simulink model "ADAC_AEBS_FailOperationTest_A3_cs"  (R2014b)
settings: Solver=ode5  SolverMode=SingleTasking  StartTime=0.0  StopTime=inf  FixedStep=1/100  RelTol=1e-3
PreLoadFcn:
  | mbxruntime.callbacks.PreLoadFcn(bdroot);
  | check_NUTS_defined;
  | 
  | assignin('base',['model_closed_' bdroot],false);addpath('../includes_AEBS');
PostLoadFcn:
  | mbxruntime.callbacks.PostLoadFcn(bdroot);
InitFcn:
  | mbxruntime.callbacks.InitFcn(bdroot);
StartFcn:
  | mbxruntime.callbacks.StartFcn(bdroot);
StopFcn:
  | mbxruntime.callbacks.StopFcn(bdroot);
model workspace: external: MAT-File .\ADAC_AEBS_FailOperationTest_A3_cs_hws.mat (data not in the file)
undefined symbols (not defined in the file or in its folder): OrientationPitch, OrientationRoll, PositionX, PositionY, PositionZ, warningInitialVelocity, x0
undefined symbols (not defined in the file): ADAC_AEBS_FailOperationTest_A3_cs_022733f5fb7b020c, ADAC_AEBS_FailOperationTest_A3_cs_0e96c704d6d8ad21, ADAC_AEBS_FailOperationTest_A3_cs_160591024d30e51e, ADAC_AEBS_FailOperationTest_A3_cs_1af48b7bc7debef8, ADAC_AEBS_FailOperationTest_A3_cs_1c8862e820c7afdc, ADAC_AEBS_FailOperationTest_A3_cs_27e9254a11318684, ADAC_AEBS_FailOperationTest_A3_cs_34a9a7fc03d9473b, ADAC_AEBS_FailOperationTest_A3_cs_530c6f2a943bd468, ADAC_AEBS_FailOperationTest_A3_cs_591c8395df5aa215, ADAC_AEBS_FailOperationTest_A3_cs_7b366378d0e5b506, ADAC_AEBS_FailOperationTest_A3_cs_7d53398e9c5959a5, ADAC_AEBS_FailOperationTest_A3_cs_943491cbf915f302, ADAC_AEBS_FailOperationTest_A3_cs_9d3d862437c23341, ADAC_AEBS_FailOperationTest_A3_cs_b6ec93f5a18de3a7, ADAC_AEBS_FailOperationTest_A3_cs_e449793b2137b4b8, SteeringColumn, SteeringWheel, WheelL0, WheelL1, WheelR0, WheelR1
libraries: simulink_extras x33, simulink x21, PreScanSimulinkLibrary x5, PreScanUsefulBlocks x2
(part 1 of 10)
CloseFcn:
  | mbxruntime.callbacks.CloseFcn(bdroot);
  | evalin('base',['clear model_closed_' bdroot]);
settings Model: Creator=PRESCAN  LastModifiedBy=jenkins
settings DataIOCC: SignalLoggingSaveFormat=ModelDataLogs
settings OptimizationCC: InlineParams=on  ExpressionDepthLimit=2147483647  InitFltsAndDblsToZero=on
settings DebuggingCC: SaveWithParameterizedLinksMsg=none  UnderspecifiedInitializationDetection=Classic  MergeDetectMultiDrivingBlocksExec=none  SignalResolutionControl=TryResolveAllWithWarning  SolverPrmCheckMsg=none  MultiTaskDSMMsg=warning  MultiTaskCondExecSysMsg=none  FcnCallInpInsideContextMsg=UseLocalSettings  StateNameClashWarn=warning
settings ModelReferenceCC: UpdateModelReferenceTargets=IfOutOfDate
settings SFSimCC: SimParseCustomCode=off
settings SFSimCC: SimCustomHeaderCode=|
  | #include "prescan.h"
  | #include "prescan_platform.h"
settings RTWCC: IncludeERTFirstTime=on
settings GRTTargetCC: TargetFcnLib=ansi_tfl_tmw.mat  CombineOutputUpdateFcns=off  GRTInterface=on

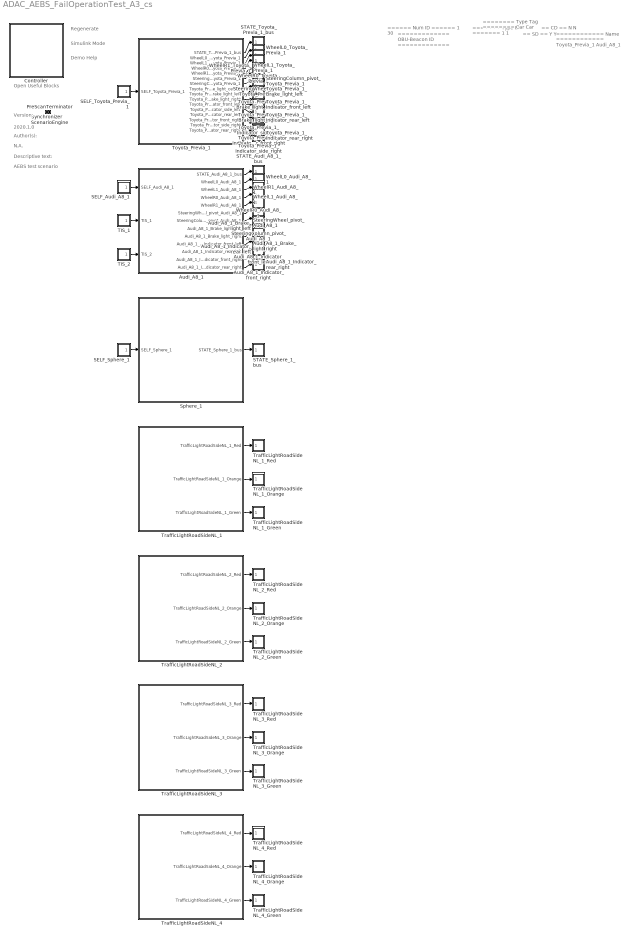
== system ADAC_AEBS_FailOperationTest_A3_cs ==
  note: Regenerate
  note: Simulink Mode
  note: Open Useful Blocks
  note: 2020.1.0
  note: Version:
  note: Author(s):
  note: N.A.
  note: Descriptive text:
  note: AEBS test scenario
  note: Demo Help
  note: ======
      | Num ID
      | ======
      | 1
      | 30
  note: =============
      | OBU-Beacon ID
      | =============
  note: =======
      | Type ID
      | =======
      | 1
      | 1
  note: ========
      | Type Tag
      | ========
      | Car
      | Car
  note: ==
      | SD
      | ==
      | Y
      | Y
  note: ==
      | CD
      | ==
      | N
      | N
  note: ============
      | Name
      | ============
      | Toyota_Previa_1
      | Audi_A8_1
  Audi_A8_1 : Subsystem  Tag=WorldObjectSubSystem  InitFcn=UniqueId = '69';
      mask init:
      | modelPath = GenericModelHelper.getGenericModelFilePath('ModelDepo','Vehicles\Audi_A8\Audi_A8.pgmb','e33fe1ddcf3e8ae97caccbc8f2fa74ac');imagePath = GenericModelHelper.getCompilationPicture(modelPath, 'Audi_A8_HighPoly.png');
      mask Display: image(imread(imagePath));color('white');text(0, 0, ' ID=30\n')
  Audi_A8_1_Brake_light_left : Subsystem  Tag=actuator/BrakeLightL  Priority=0  LoadFcn=load('PreScanVisuLightActuatorData');load('PrescanRPYData');load('PrescanXYZData');load('PreScanRGBData')  mask(PreScan Sink Block: VisuActiveLight){}
      mask help:
      | The VisuActiveLight block provides a way for detailed animation of Light Sources, such as the indicator, brake, fog and main lights of a vehicle, or a light post.
      |
      | For more information, please click Help.
      settings: OpenFcn=open_system([gcb '/Actuator'],'mask')
      mask Help: eval('openHelp(209)')
      mask Display: image(imread('HeadLight.png'))
  Audi_A8_1_Brake_light_right : Subsystem  Tag=actuator/BrakeLightR  Priority=0  LoadFcn=load('PreScanVisuLightActuatorData');load('PrescanRPYData');load('PrescanXYZData');load('PreScanRGBData')  mask(PreScan Sink Block: VisuActiveLight){}
      mask help:
      | The VisuActiveLight block provides a way for detailed animation of Light Sources, such as the indicator, brake, fog and main lights of a vehicle, or a light post.
      |
      | For more information, please click Help.
      settings: OpenFcn=open_system([gcb '/Actuator'],'mask')
      mask Help: eval('openHelp(209)')
      mask Display: image(imread('HeadLight.png'))
  Audi_A8_1_Indicator_front_left : Subsystem  Tag=actuator/IndicatorFL  Priority=0  LoadFcn=load('PreScanVisuLightActuatorData');load('PrescanRPYData');load('PrescanXYZData');load('PreScanRGBData')  mask(PreScan Sink Block: VisuActiveLight){}
      mask help:
      | The VisuActiveLight block provides a way for detailed animation of Light Sources, such as the indicator, brake, fog and main lights of a vehicle, or a light post.
      |
      | For more information, please click Help.
      settings: OpenFcn=open_system([gcb '/Actuator'],'mask')
      mask Help: eval('openHelp(209)')
      mask Display: image(imread('HeadLight.png'))
  Audi_A8_1_Indicator_front_right : Subsystem  Tag=actuator/IndicatorFR  Priority=0  LoadFcn=load('PreScanVisuLightActuatorData');load('PrescanRPYData');load('PrescanXYZData');load('PreScanRGBData')  mask(PreScan Sink Block: VisuActiveLight){}
      mask help:
      | The VisuActiveLight block provides a way for detailed animation of Light Sources, such as the indicator, brake, fog and main lights of a vehicle, or a light post.
      |
      | For more information, please click Help.
      settings: OpenFcn=open_system([gcb '/Actuator'],'mask')
      mask Help: eval('openHelp(209)')
      mask Display: image(imread('HeadLight.png'))
  Audi_A8_1_Indicator_rear_left : Subsystem  Tag=actuator/IndicatorRL  Priority=0  LoadFcn=load('PreScanVisuLightActuatorData');load('PrescanRPYData');load('PrescanXYZData');load('PreScanRGBData')  mask(PreScan Sink Block: VisuActiveLight){}
      mask help:
      | The VisuActiveLight block provides a way for detailed animation of Light Sources, such as the indicator, brake, fog and main lights of a vehicle, or a light post.
      |
      | For more information, please click Help.
      settings: OpenFcn=open_system([gcb '/Actuator'],'mask')
      mask Help: eval('openHelp(209)')
      mask Display: image(imread('HeadLight.png'))
  Audi_A8_1_Indicator_rear_right : Subsystem  Tag=actuator/IndicatorRR  Priority=0  LoadFcn=load('PreScanVisuLightActuatorData');load('PrescanRPYData');load('PrescanXYZData');load('PreScanRGBData')  mask(PreScan Sink Block: VisuActiveLight){}
      mask help:
      | The VisuActiveLight block provides a way for detailed animation of Light Sources, such as the indicator, brake, fog and main lights of a vehicle, or a light post.
      |
      | For more information, please click Help.
      settings: OpenFcn=open_system([gcb '/Actuator'],'mask')
      mask Help: eval('openHelp(209)')
      mask Display: image(imread('HeadLight.png'))
  Controller : Subsystem  Description=8A3CD2955739A82C886C20AE3E253D78460D53180EE2C1B14CC08DF75A70BE77  Priority=-1  LoadFcn=load PreScanControllerData  mask(PreScan Simulation Controller){prescanversion='2020.1.0', ModelReferencing=off, TimeStep=1/100, ControlMode=0, PreScanExecutionMode=on, ControllerCount=0, ControllerIndex=0, ControllerOptions=''}
      mask prompts: prescanversion "PreScan Version"; ModelReferencing "Use Model Referencing"; TimeStep "Upload Period [s]"; ControlMode "Control Mode"; PreScanExecutionMode "Execution Mode"; ControllerCount "Controller Count"; ControllerIndex "Controller Index"; ControllerOptions "Controller Options"
      mask help:
      | Please do not remove this block from the compilation sheet,
      | as it connects the model to the PreScan environment.
      mask init:
      | model = bdroot(gcb);
      | ExperimentFile = mbxruntime.findExperimentFile(model,true); %relative path
      | 
      | [d1, d2, d3, prescandata] = prescan_Settings();
      | ModelDepo = fullfile(prescandata,'ModelDepo'); 
      | 
      | RTmode = mbxruntime.getRTMode(model);
      | 
      | SimulationMode = get_param(bdroot,'SimulationMode');
      | if strcmp(SimulationMode, 'rapid-accelerator')
      |     SimulationMode = 'external';
      | end
      | TargetName = get_param(bdroot,'SystemTargetFile');
      settings: ModelCloseFcn=assignin('base',['model_closed_' bdroot],true);
      mask Help: eval('openHelp(812)')
      mask Display: image(imread('prescanlogo.ico'))
  PreScanTerminator : Subsystem  Tag=PreScanTerminator  Priority=999  LoadFcn=load PrescanTerminatorData  mask(PreScan Simulation Terminator){TimeStep=1/100}
      mask prompts: TimeStep "Upload Period [s]"
      mask help:
      | Please do not remove this block from the compilation sheet as it
      | connects the model to the PreScan environment.
      mask Help: eval('openHelp(812)')
      mask Display: image(imread('prescanlogo.ico'))
  SELF_Audi_A8_1 : Subsystem  Tag=sensor/SelfPort  Priority=30  LoadFcn=load('PreScanSelfSensorData.mat')  mask(PreScan Source Block: SELF){}
      mask help:
      | The SELF port shows (state) information of the actor itself. The outputs are position in the experiment's axis system and the GPS coordinates, and the object's absolute velocity and compass heading.
      |
      | For more information, please click Help.
      settings: OpenFcn=open_system([gcb '/Sensor'],'mask')
      mask Help: eval('openHelp(462)')
      mask Display: image(imread('GPS.png'))
  SELF_Sphere_1 : Subsystem  Tag=sensor/SelfPort  Priority=30  LoadFcn=load('PreScanSelfSensorData.mat')  mask(PreScan Source Block: SELF){}
      mask help:
      | The SELF port shows (state) information of the actor itself. The outputs are position in the experiment's axis system and the GPS coordinates, and the object's absolute velocity and compass heading.
      |
      | For more information, please click Help.
      settings: OpenFcn=open_system([gcb '/Sensor'],'mask')
      mask Help: eval('openHelp(462)')
      mask Display: image(imread('GPS.png'))
  SELF_Toyota_Previa_1 : Subsystem  Tag=sensor/SelfPort  Priority=30  LoadFcn=load('PreScanSelfSensorData.mat')  mask(PreScan Source Block: SELF){}
      mask help:
      | The SELF port shows (state) information of the actor itself. The outputs are position in the experiment's axis system and the GPS coordinates, and the object's absolute velocity and compass heading.
      |
      | For more information, please click Help.
      settings: OpenFcn=open_system([gcb '/Sensor'],'mask')
      mask Help: eval('openHelp(462)')
      mask Display: image(imread('GPS.png'))
  STATE_Audi_A8_1_bus : Subsystem  Tag=actuator/StatePort  Priority=0  LoadFcn=load('PreScanStateActuatorData.mat')  mask(PreScan Sink Block: State){}
      mask help:
      | The Actor State contains a vector signal of size (9x1), containing the following signals:
      |
      | -  Position    	(x,y,z)             	[m]
      | -  Velocity    	(vx,vy,vz)         	[m/s]
      | -  Angles       	(Roll, Pitch, Yaw)	[rad]
      |
      | The Actor state is defined in the global axis system.
      | The state is superponed on the Initial position defined in the GUI.
      |
      | For more information, please click Help.
      settings: OpenFcn=open_system([gcb '/Actuator'],'mask')
      mask Help: eval('openHelp(222)')
      mask Display: image(imread('State.png'))
  STATE_Sphere_1_bus : Subsystem  Tag=actuator/StatePort  Priority=0  LoadFcn=load('PreScanStateActuatorData.mat')  mask(PreScan Sink Block: State){}
      mask help:
      | The Actor State contains a vector signal of size (9x1), containing the following signals:
      |
      | -  Position    	(x,y,z)             	[m]
      | -  Velocity    	(vx,vy,vz)         	[m/s]
      | -  Angles       	(Roll, Pitch, Yaw)	[rad]
      |
      | The Actor state is defined in the global axis system.
      | The state is superponed on the Initial position defined in the GUI.
      |
      | For more information, please click Help.
      settings: OpenFcn=open_system([gcb '/Actuator'],'mask')
      mask Help: eval('openHelp(222)')
      mask Display: image(imread('State.png'))
  STATE_Toyota_Previa_1_bus : Subsystem  Tag=actuator/StatePort  Priority=0  LoadFcn=load('PreScanStateActuatorData.mat')  mask(PreScan Sink Block: State){}
      mask help:
      | The Actor State contains a vector signal of size (9x1), containing the following signals:
      |
      | -  Position    	(x,y,z)             	[m]
      | -  Velocity    	(vx,vy,vz)         	[m/s]
      | -  Angles       	(Roll, Pitch, Yaw)	[rad]
      |
      | The Actor state is defined in the global axis system.
      | The state is superponed on the Initial position defined in the GUI.
      |
      | For more information, please click Help.
      settings: OpenFcn=open_system([gcb '/Actuator'],'mask')
      mask Help: eval('openHelp(222)')
      mask Display: image(imread('State.png'))
  ScenarioEngine : Subsystem  Tag=PreScanOpenScenarioBlock  Priority=10  LoadFcn=load PrescanSynchronizeData  mask(PreScan Simulation Core Block){TimeStep=1/100}
      mask prompts: TimeStep "Timestep [s]"
      mask help:
      | Please do not remove this block from the PreScan compilation sheet,
      | as it contains essential configuration parameters for a PreScan simulation.
      settings: DeleteFcn=PreScanBlockDeleteFcn;
      mask Display: image(imread('prescanlogo.ico'))
  Sphere_1 : Subsystem  Tag=WorldObjectSubSystem  InitFcn=UniqueId = '77';
      mask init:
      | imagePath=which('Sphere.jpg');
      mask Display: image(imread(imagePath));color('white');text(0, 0, ' ID=7\n')
  SteeringColumn_pivot_Audi_A8_1 : Subsystem  Tag=Actuator  Priority=0  LoadFcn=load('PrescanPoseData');load('PrescanXYZData');load('PreScanRPYData')
      mask help:
      | The VisuJoint block provides a way to adapt the location and orientation of a part of an object.
      |
      | For more information, please click Help.
      settings: OpenFcn=open_system([gcb '/Actuator'],'mask')
      mask Display: image(imread('Joint.png'))
  SteeringColumn_pivot_Toyota_Previa_1 : Subsystem  Tag=Actuator  Priority=0  LoadFcn=load('PrescanPoseData');load('PrescanXYZData');load('PreScanRPYData')
      mask help:
      | The VisuJoint block provides a way to adapt the location and orientation of a part of an object.
      |
      | For more information, please click Help.
      settings: OpenFcn=open_system([gcb '/Actuator'],'mask')
      mask Display: image(imread('Joint.png'))
  SteeringWheel_pivot_Audi_A8_1 : Subsystem  Tag=Actuator  Priority=0  LoadFcn=load('PrescanPoseData');load('PrescanXYZData');load('PreScanRPYData')
      mask help:
      | The VisuJoint block provides a way to adapt the location and orientation of a part of an object.
      |
      | For more information, please click Help.
      settings: OpenFcn=open_system([gcb '/Actuator'],'mask')
      mask Display: image(imread('Joint.png'))
  SteeringWheel_pivot_Toyota_Previa_1 : Subsystem  Tag=Actuator  Priority=0  LoadFcn=load('PrescanPoseData');load('PrescanXYZData');load('PreScanRPYData')
      mask help:
      | The VisuJoint block provides a way to adapt the location and orientation of a part of an object.
      |
      | For more information, please click Help.
      settings: OpenFcn=open_system([gcb '/Actuator'],'mask')
      mask Display: image(imread('Joint.png'))
  Synchronizer : Subsystem  Tag=PreScanSynchronizer  Priority=20  LoadFcn=load PrescanSynchronizeData  mask(PreScan Simulation Core Block){TimeStep=1/100}
      mask prompts: TimeStep "Timestep [s]"
      mask help:
      | Please do not remove this block from the PreScan compilation sheet,
      | as it contains essential configuration parameters for a PreScan simulation.
      settings: DeleteFcn=PreScanBlockDeleteFcn;
      mask Display: image(imread('prescanlogo.ico'))
  TIS_1 : Subsystem  Tag=sensor/TIS  Priority=30  LoadFcn=load('PrescanScannerSensorData.mat');load('PrescanScannerSensorMessage.mat')  mask(PreScan Source Block: Technology Independent Sensor (TIS)){}
      mask help:
      | The Technology Independent Sensor (TIS) provides a sensor with all sensor-related influence factors (like noise, drift and accuracy) without being technology specific (like radar and lidar). The TIS detects the closest point on the geometry of an object.
      |
      | For more information, please click Help.
      settings: OpenFcn=open_system([gcb '/Sensor'],'mask')
      mask Help: eval('openHelp(449)')
      mask Display: image(imread('TIS.png'))
  TIS_2 : Subsystem  Tag=sensor/TIS  Priority=30  LoadFcn=load('PrescanScannerSensorData.mat');load('PrescanScannerSensorMessage.mat')  mask(PreScan Source Block: Technology Independent Sensor (TIS)){}
      mask help:
      | The Technology Independent Sensor (TIS) provides a sensor with all sensor-related influence factors (like noise, drift and accuracy) without being technology specific (like radar and lidar). The TIS detects the closest point on the geometry of an object.
      |
      | For more information, please click Help.
      settings: OpenFcn=open_system([gcb '/Sensor'],'mask')
      mask Help: eval('openHelp(449)')
      mask Display: image(imread('TIS.png'))
  Toyota_Previa_1 : Subsystem  Tag=WorldObjectSubSystem  InitFcn=UniqueId = '17';
      mask init:
      | modelPath = GenericModelHelper.getGenericModelFilePath('ModelDepo','Vehicles\Toyota_Previa\Toyota_Previa.pgmb','93e58f95175b34f6ce91a88cdfe55b40');imagePath = GenericModelHelper.getCompilationPicture(modelPath, 'Toyota_Previa_HighPoly.png');
      mask Display: image(imread(imagePath));color('white');text(0, 0, ' ID=1\n')
  Toyota_Previa_1_Brake_light_center : Subsystem  Tag=actuator/BrakeLightM  Priority=0  LoadFcn=load('PreScanVisuLightActuatorData');load('PrescanRPYData');load('PrescanXYZData');load('PreScanRGBData')  mask(PreScan Sink Block: VisuActiveLight){}
      mask help:
      | The VisuActiveLight block provides a way for detailed animation of Light Sources, such as the indicator, brake, fog and main lights of a vehicle, or a light post.
      |
      | For more information, please click Help.
      settings: OpenFcn=open_system([gcb '/Actuator'],'mask')
      mask Help: eval('openHelp(209)')
      mask Display: image(imread('HeadLight.png'))
  Toyota_Previa_1_Brake_light_left : Subsystem  Tag=actuator/BrakeLightL  Priority=0  LoadFcn=load('PreScanVisuLightActuatorData');load('PrescanRPYData');load('PrescanXYZData');load('PreScanRGBData')  mask(PreScan Sink Block: VisuActiveLight){}
      mask help:
      | The VisuActiveLight block provides a way for detailed animation of Light Sources, such as the indicator, brake, fog and main lights of a vehicle, or a light post.
      |
      | For more information, please click Help.
      settings: OpenFcn=open_system([gcb '/Actuator'],'mask')
      mask Help: eval('openHelp(209)')
      mask Display: image(imread('HeadLight.png'))
  Toyota_Previa_1_Brake_light_right : Subsystem  Tag=actuator/BrakeLightR  Priority=0  LoadFcn=load('PreScanVisuLightActuatorData');load('PrescanRPYData');load('PrescanXYZData');load('PreScanRGBData')  mask(PreScan Sink Block: VisuActiveLight){}
      mask help:
      | The VisuActiveLight block provides a way for detailed animation of Light Sources, such as the indicator, brake, fog and main lights of a vehicle, or a light post.
      |
      | For more information, please click Help.
      settings: OpenFcn=open_system([gcb '/Actuator'],'mask')
      mask Help: eval('openHelp(209)')
      mask Display: image(imread('HeadLight.png'))
  Toyota_Previa_1_Indicator_front_left : Subsystem  Tag=actuator/IndicatorFL  Priority=0  LoadFcn=load('PreScanVisuLightActuatorData');load('PrescanRPYData');load('PrescanXYZData');load('PreScanRGBData')  mask(PreScan Sink Block: VisuActiveLight){}
      mask help:
      | The VisuActiveLight block provides a way for detailed animation of Light Sources, such as the indicator, brake, fog and main lights of a vehicle, or a light post.
      |
      | For more information, please click Help.
      settings: OpenFcn=open_system([gcb '/Actuator'],'mask')
      mask Help: eval('openHelp(209)')
      mask Display: image(imread('HeadLight.png'))
  Toyota_Previa_1_Indicator_front_right : Subsystem  Tag=actuator/IndicatorFR  Priority=0  LoadFcn=load('PreScanVisuLightActuatorData');load('PrescanRPYData');load('PrescanXYZData');load('PreScanRGBData')  mask(PreScan Sink Block: VisuActiveLight){}
      mask help:
      | The VisuActiveLight block provides a way for detailed animation of Light Sources, such as the indicator, brake, fog and main lights of a vehicle, or a light post.
      |
      | For more information, please click Help.
      settings: OpenFcn=open_system([gcb '/Actuator'],'mask')
      mask Help: eval('openHelp(209)')
      mask Display: image(imread('HeadLight.png'))
  Toyota_Previa_1_Indicator_rear_left : Subsystem  Tag=actuator/IndicatorRL  Priority=0  LoadFcn=load('PreScanVisuLightActuatorData');load('PrescanRPYData');load('PrescanXYZData');load('PreScanRGBData')  mask(PreScan Sink Block: VisuActiveLight){}
      mask help:
      | The VisuActiveLight block provides a way for detailed animation of Light Sources, such as the indicator, brake, fog and main lights of a vehicle, or a light post.
      |
      | For more information, please click Help.
      settings: OpenFcn=open_system([gcb '/Actuator'],'mask')
      mask Help: eval('openHelp(209)')
      mask Display: image(imread('HeadLight.png'))
  Toyota_Previa_1_Indicator_rear_right : Subsystem  Tag=actuator/IndicatorRR  Priority=0  LoadFcn=load('PreScanVisuLightActuatorData');load('PrescanRPYData');load('PrescanXYZData');load('PreScanRGBData')  mask(PreScan Sink Block: VisuActiveLight){}
      mask help:
      | The VisuActiveLight block provides a way for detailed animation of Light Sources, such as the indicator, brake, fog and main lights of a vehicle, or a light post.
      |
      | For more information, please click Help.
      settings: OpenFcn=open_system([gcb '/Actuator'],'mask')
      mask Help: eval('openHelp(209)')
      mask Display: image(imread('HeadLight.png'))
  Toyota_Previa_1_Indicator_side_left : Subsystem  Tag=actuator/IndicatorSL  Priority=0  LoadFcn=load('PreScanVisuLightActuatorData');load('PrescanRPYData');load('PrescanXYZData');load('PreScanRGBData')  mask(PreScan Sink Block: VisuActiveLight){}
      mask help:
      | The VisuActiveLight block provides a way for detailed animation of Light Sources, such as the indicator, brake, fog and main lights of a vehicle, or a light post.
      |
      | For more information, please click Help.
      settings: OpenFcn=open_system([gcb '/Actuator'],'mask')
      mask Help: eval('openHelp(209)')
      mask Display: image(imread('HeadLight.png'))
  Toyota_Previa_1_Indicator_side_right : Subsystem  Tag=actuator/IndicatorSR  Priority=0  LoadFcn=load('PreScanVisuLightActuatorData');load('PrescanRPYData');load('PrescanXYZData');load('PreScanRGBData')  mask(PreScan Sink Block: VisuActiveLight){}
      mask help:
      | The VisuActiveLight block provides a way for detailed animation of Light Sources, such as the indicator, brake, fog and main lights of a vehicle, or a light post.
      |
      | For more information, please click Help.
      settings: OpenFcn=open_system([gcb '/Actuator'],'mask')
      mask Help: eval('openHelp(209)')
      mask Display: image(imread('HeadLight.png'))
  TrafficLightRoadSideNL_1 : Subsystem  Tag=WorldObjectSubSystem  InitFcn=UniqueId = '42';
      mask init:
      | modelPath = GenericModelHelper.getGenericModelFilePath('ModelDepo','AnimatedElements\TrafficLight_NL\Roadside\Roadside_NL.pgmb','2000fba5e1a6d0fba32e88146243c3cb');imagePath = GenericModelHelper.getCompilationPicture(modelPath, 'Roadside_NL.png');
      mask Display: image(imread(imagePath));color('white');text(0, 0, ' ID=14\n')
  TrafficLightRoadSideNL_1_Green : Subsystem  Tag=actuator/Green  Priority=0  LoadFcn=load('PreScanVisuLightActuatorData');load('PrescanRPYData');load('PrescanXYZData');load('PreScanRGBData')  mask(PreScan Sink Block: VisuActiveLight){}
      mask help:
      | The VisuActiveLight block provides a way for detailed animation of Light Sources, such as the indicator, brake, fog and main lights of a vehicle, or a light post.
      |
      | For more information, please click Help.
      settings: OpenFcn=open_system([gcb '/Actuator'],'mask')
      mask Help: eval('openHelp(209)')
      mask Display: image(imread('HeadLight.png'))
  TrafficLightRoadSideNL_1_Orange : Subsystem  Tag=actuator/Orange  Priority=0  LoadFcn=load('PreScanVisuLightActuatorData');load('PrescanRPYData');load('PrescanXYZData');load('PreScanRGBData')  mask(PreScan Sink Block: VisuActiveLight){}
      mask help:
      | The VisuActiveLight block provides a way for detailed animation of Light Sources, such as the indicator, brake, fog and main lights of a vehicle, or a light post.
      |
      | For more information, please click Help.
      settings: OpenFcn=open_system([gcb '/Actuator'],'mask')
      mask Help: eval('openHelp(209)')
      mask Display: image(imread('HeadLight.png'))
  TrafficLightRoadSideNL_1_Red : Subsystem  Tag=actuator/Red  Priority=0  LoadFcn=load('PreScanVisuLightActuatorData');load('PrescanRPYData');load('PrescanXYZData');load('PreScanRGBData')  mask(PreScan Sink Block: VisuActiveLight){}
      mask help:
      | The VisuActiveLight block provides a way for detailed animation of Light Sources, such as the indicator, brake, fog and main lights of a vehicle, or a light post.
      |
      | For more information, please click Help.
      settings: OpenFcn=open_system([gcb '/Actuator'],'mask')
      mask Help: eval('openHelp(209)')
      mask Display: image(imread('HeadLight.png'))
  TrafficLightRoadSideNL_2 : Subsystem  Tag=WorldObjectSubSystem  InitFcn=UniqueId = '43';
      mask init: same as ADAC_AEBS_FailOperationTest_A3_cs/TrafficLightRoadSideNL_1
      mask Display: image(imread(imagePath));color('white');text(0, 0, ' ID=21\n')
  TrafficLightRoadSideNL_2_Green : Subsystem  Tag=actuator/Green  Priority=0  LoadFcn=load('PreScanVisuLightActuatorData');load('PrescanRPYData');load('PrescanXYZData');load('PreScanRGBData')  mask(PreScan Sink Block: VisuActiveLight){}
      mask help:
      | The VisuActiveLight block provides a way for detailed animation of Light Sources, such as the indicator, brake, fog and main lights of a vehicle, or a light post.
      |
      | For more information, please click Help.
      settings: OpenFcn=open_system([gcb '/Actuator'],'mask')
      mask Help: eval('openHelp(209)')
      mask Display: image(imread('HeadLight.png'))
  TrafficLightRoadSideNL_2_Orange : Subsystem  Tag=actuator/Orange  Priority=0  LoadFcn=load('PreScanVisuLightActuatorData');load('PrescanRPYData');load('PrescanXYZData');load('PreScanRGBData')  mask(PreScan Sink Block: VisuActiveLight){}
      mask help:
      | The VisuActiveLight block provides a way for detailed animation of Light Sources, such as the indicator, brake, fog and main lights of a vehicle, or a light post.
      |
      | For more information, please click Help.
      settings: OpenFcn=open_system([gcb '/Actuator'],'mask')
      mask Help: eval('openHelp(209)')
      mask Display: image(imread('HeadLight.png'))
  TrafficLightRoadSideNL_2_Red : Subsystem  Tag=actuator/Red  Priority=0  LoadFcn=load('PreScanVisuLightActuatorData');load('PrescanRPYData');load('PrescanXYZData');load('PreScanRGBData')  mask(PreScan Sink Block: VisuActiveLight){}
      mask help:
      | The VisuActiveLight block provides a way for detailed animation of Light Sources, such as the indicator, brake, fog and main lights of a vehicle, or a light post.
      |
      | For more information, please click Help.
      settings: OpenFcn=open_system([gcb '/Actuator'],'mask')
      mask Help: eval('openHelp(209)')
      mask Display: image(imread('HeadLight.png'))
  TrafficLightRoadSideNL_3 : Subsystem  Tag=WorldObjectSubSystem  InitFcn=UniqueId = '44';
      mask init: same as ADAC_AEBS_FailOperationTest_A3_cs/TrafficLightRoadSideNL_1
      mask Display: image(imread(imagePath));color('white');text(0, 0, ' ID=22\n')
  TrafficLightRoadSideNL_3_Green : Subsystem  Tag=actuator/Green  Priority=0  LoadFcn=load('PreScanVisuLightActuatorData');load('PrescanRPYData');load('PrescanXYZData');load('PreScanRGBData')  mask(PreScan Sink Block: VisuActiveLight){}
      mask help:
      | The VisuActiveLight block provides a way for detailed animation of Light Sources, such as the indicator, brake, fog and main lights of a vehicle, or a light post.
      |
      | For more information, please click Help.
      settings: OpenFcn=open_system([gcb '/Actuator'],'mask')
      mask Help: eval('openHelp(209)')
      mask Display: image(imread('HeadLight.png'))
  TrafficLightRoadSideNL_3_Orange : Subsystem  Tag=actuator/Orange  Priority=0  LoadFcn=load('PreScanVisuLightActuatorData');load('PrescanRPYData');load('PrescanXYZData');load('PreScanRGBData')  mask(PreScan Sink Block: VisuActiveLight){}
      mask help:
      | The VisuActiveLight block provides a way for detailed animation of Light Sources, such as the indicator, brake, fog and main lights of a vehicle, or a light post.
      |
      | For more information, please click Help.
      settings: OpenFcn=open_system([gcb '/Actuator'],'mask')
      mask Help: eval('openHelp(209)')
      mask Display: image(imread('HeadLight.png'))
  TrafficLightRoadSideNL_3_Red : Subsystem  Tag=actuator/Red  Priority=0  LoadFcn=load('PreScanVisuLightActuatorData');load('PrescanRPYData');load('PrescanXYZData');load('PreScanRGBData')  mask(PreScan Sink Block: VisuActiveLight){}
      mask help:
      | The VisuActiveLight block provides a way for detailed animation of Light Sources, such as the indicator, brake, fog and main lights of a vehicle, or a light post.
      |
      | For more information, please click Help.
      settings: OpenFcn=open_system([gcb '/Actuator'],'mask')
      mask Help: eval('openHelp(209)')
      mask Display: image(imread('HeadLight.png'))
  TrafficLightRoadSideNL_4 : Subsystem  Tag=WorldObjectSubSystem  InitFcn=UniqueId = '45';
      mask init: same as ADAC_AEBS_FailOperationTest_A3_cs/TrafficLightRoadSideNL_1
      mask Display: image(imread(imagePath));color('white');text(0, 0, ' ID=23\n')
  TrafficLightRoadSideNL_4_Green : Subsystem  Tag=actuator/Green  Priority=0  LoadFcn=load('PreScanVisuLightActuatorData');load('PrescanRPYData');load('PrescanXYZData');load('PreScanRGBData')  mask(PreScan Sink Block: VisuActiveLight){}
      mask help:
      | The VisuActiveLight block provides a way for detailed animation of Light Sources, such as the indicator, brake, fog and main lights of a vehicle, or a light post.
      |
      | For more information, please click Help.
      settings: OpenFcn=open_system([gcb '/Actuator'],'mask')
      mask Help: eval('openHelp(209)')
      mask Display: image(imread('HeadLight.png'))
  TrafficLightRoadSideNL_4_Orange : Subsystem  Tag=actuator/Orange  Priority=0  LoadFcn=load('PreScanVisuLightActuatorData');load('PrescanRPYData');load('PrescanXYZData');load('PreScanRGBData')  mask(PreScan Sink Block: VisuActiveLight){}
      mask help:
      | The VisuActiveLight block provides a way for detailed animation of Light Sources, such as the indicator, brake, fog and main lights of a vehicle, or a light post.
      |
      | For more information, please click Help.
      settings: OpenFcn=open_system([gcb '/Actuator'],'mask')
      mask Help: eval('openHelp(209)')
      mask Display: image(imread('HeadLight.png'))
  TrafficLightRoadSideNL_4_Red : Subsystem  Tag=actuator/Red  Priority=0  LoadFcn=load('PreScanVisuLightActuatorData');load('PrescanRPYData');load('PrescanXYZData');load('PreScanRGBData')  mask(PreScan Sink Block: VisuActiveLight){}
      mask help:
      | The VisuActiveLight block provides a way for detailed animation of Light Sources, such as the indicator, brake, fog and main lights of a vehicle, or a light post.
      |
      | For more information, please click Help.
      settings: OpenFcn=open_system([gcb '/Actuator'],'mask')
      mask Help: eval('openHelp(209)')
      mask Display: image(imread('HeadLight.png'))
  WheelL0_Audi_A8_1 : Subsystem  Tag=Actuator  Priority=0  LoadFcn=load('PrescanPoseData');load('PrescanXYZData');load('PreScanRPYData')
      mask help:
      | The VisuJoint block provides a way to adapt the location and orientation of a part of an object.
      |
      | For more information, please click Help.
      settings: OpenFcn=open_system([gcb '/Actuator'],'mask')
      mask Display: image(imread('Joint.png'))
  WheelL0_Toyota_Previa_1 : Subsystem  Tag=Actuator  Priority=0  LoadFcn=load('PrescanPoseData');load('PrescanXYZData');load('PreScanRPYData')
      mask help:
      | The VisuJoint block provides a way to adapt the location and orientation of a part of an object.
      |
      | For more information, please click Help.
      settings: OpenFcn=open_system([gcb '/Actuator'],'mask')
      mask Display: image(imread('Joint.png'))
  WheelL1_Audi_A8_1 : Subsystem  Tag=Actuator  Priority=0  LoadFcn=load('PrescanPoseData');load('PrescanXYZData');load('PreScanRPYData')
      mask help:
      | The VisuJoint block provides a way to adapt the location and orientation of a part of an object.
      |
      | For more information, please click Help.
      settings: OpenFcn=open_system([gcb '/Actuator'],'mask')
      mask Display: image(imread('Joint.png'))
  WheelL1_Toyota_Previa_1 : Subsystem  Tag=Actuator  Priority=0  LoadFcn=load('PrescanPoseData');load('PrescanXYZData');load('PreScanRPYData')
      mask help:
      | The VisuJoint block provides a way to adapt the location and orientation of a part of an object.
      |
      | For more information, please click Help.
      settings: OpenFcn=open_system([gcb '/Actuator'],'mask')
      mask Display: image(imread('Joint.png'))
  WheelR0_Audi_A8_1 : Subsystem  Tag=Actuator  Priority=0  LoadFcn=load('PrescanPoseData');load('PrescanXYZData');load('PreScanRPYData')
      mask help:
      | The VisuJoint block provides a way to adapt the location and orientation of a part of an object.
      |
      | For more information, please click Help.
      settings: OpenFcn=open_system([gcb '/Actuator'],'mask')
      mask Display: image(imread('Joint.png'))
  WheelR0_Toyota_Previa_1 : Subsystem  Tag=Actuator  Priority=0  LoadFcn=load('PrescanPoseData');load('PrescanXYZData');load('PreScanRPYData')
      mask help:
      | The VisuJoint block provides a way to adapt the location and orientation of a part of an object.
      |
      | For more information, please click Help.
      settings: OpenFcn=open_system([gcb '/Actuator'],'mask')
      mask Display: image(imread('Joint.png'))
  WheelR1_Audi_A8_1 : Subsystem  Tag=Actuator  Priority=0  LoadFcn=load('PrescanPoseData');load('PrescanXYZData');load('PreScanRPYData')
      mask help:
      | The VisuJoint block provides a way to adapt the location and orientation of a part of an object.
      |
      | For more information, please click Help.
      settings: OpenFcn=open_system([gcb '/Actuator'],'mask')
      mask Display: image(imread('Joint.png'))
  WheelR1_Toyota_Previa_1 : Subsystem  Tag=Actuator  Priority=0  LoadFcn=load('PrescanPoseData');load('PrescanXYZData');load('PreScanRPYData')
      mask help:
      | The VisuJoint block provides a way to adapt the location and orientation of a part of an object.
      |
      | For more information, please click Help.
      settings: OpenFcn=open_system([gcb '/Actuator'],'mask')
      mask Display: image(imread('Joint.png'))
  wires:
  Toyota_Previa_1/1(STATE_Toyota_Previa_1_bus) -> STATE_Toyota_Previa_1_bus/1(STATE_Toyota_Previa_1_bus)
  SELF_Toyota_Previa_1/1(SELF_Toyota_Previa_1) -> Toyota_Previa_1/1(SELF_Toyota_Previa_1)
  Toyota_Previa_1/2(WheelL0_Toyota_Previa_1) -> WheelL0_Toyota_Previa_1/1(WheelL0_Toyota_Previa_1)
  Toyota_Previa_1/3(WheelL1_Toyota_Previa_1) -> WheelL1_Toyota_Previa_1/1(WheelL1_Toyota_Previa_1)
  Toyota_Previa_1/4(WheelR0_Toyota_Previa_1) -> WheelR0_Toyota_Previa_1/1(WheelR0_Toyota_Previa_1)
  Toyota_Previa_1/5(WheelR1_Toyota_Previa_1) -> WheelR1_Toyota_Previa_1/1(WheelR1_Toyota_Previa_1)
  Toyota_Previa_1/6(SteeringWheel_pivot_Toyota_Previa_1) -> SteeringWheel_pivot_Toyota_Previa_1/1(SteeringWheel_pivot_Toyota_Previa_1)
  Toyota_Previa_1/7(SteeringColumn_pivot_Toyota_Previa_1) -> SteeringColumn_pivot_Toyota_Previa_1/1(SteeringColumn_pivot_Toyota_Previa_1)
  Toyota_Previa_1/8(Toyota_Previa_1_Brake_light_center) -> Toyota_Previa_1_Brake_light_center/1(Toyota_Previa_1_Brake_light_center)
  Toyota_Previa_1/9(Toyota_Previa_1_Brake_light_left) -> Toyota_Previa_1_Brake_light_left/1(Toyota_Previa_1_Brake_light_left)
  Toyota_Previa_1/10(Toyota_Previa_1_Brake_light_right) -> Toyota_Previa_1_Brake_light_right/1(Toyota_Previa_1_Brake_light_right)
  Toyota_Previa_1/11(Toyota_Previa_1_Indicator_front_left) -> Toyota_Previa_1_Indicator_front_left/1(Toyota_Previa_1_Indicator_front_left)
  Toyota_Previa_1/12(Toyota_Previa_1_Indicator_side_left) -> Toyota_Previa_1_Indicator_side_left/1(Toyota_Previa_1_Indicator_side_left)
  Toyota_Previa_1/13(Toyota_Previa_1_Indicator_rear_left) -> Toyota_Previa_1_Indicator_rear_left/1(Toyota_Previa_1_Indicator_rear_left)
  Toyota_Previa_1/14(Toyota_Previa_1_Indicator_front_right) -> Toyota_Previa_1_Indicator_front_right/1(Toyota_Previa_1_Indicator_front_right)
  Toyota_Previa_1/15(Toyota_Previa_1_Indicator_side_right) -> Toyota_Previa_1_Indicator_side_right/1(Toyota_Previa_1_Indicator_side_right)
  Toyota_Previa_1/16(Toyota_Previa_1_Indicator_rear_right) -> Toyota_Previa_1_Indicator_rear_right/1(Toyota_Previa_1_Indicator_rear_right)
  Audi_A8_1/1(STATE_Audi_A8_1_bus) -> STATE_Audi_A8_1_bus/1(STATE_Audi_A8_1_bus)
  SELF_Audi_A8_1/1(SELF_Audi_A8_1) -> Audi_A8_1/1(SELF_Audi_A8_1)
  TIS_1/1(TIS_1) -> Audi_A8_1/2(TIS_1)
  TIS_2/1(TIS_2) -> Audi_A8_1/3(TIS_2)
  Audi_A8_1/2(WheelL0_Audi_A8_1) -> WheelL0_Audi_A8_1/1(WheelL0_Audi_A8_1)
  Audi_A8_1/3(WheelL1_Audi_A8_1) -> WheelL1_Audi_A8_1/1(WheelL1_Audi_A8_1)
  Audi_A8_1/4(WheelR0_Audi_A8_1) -> WheelR0_Audi_A8_1/1(WheelR0_Audi_A8_1)
  Audi_A8_1/5(WheelR1_Audi_A8_1) -> WheelR1_Audi_A8_1/1(WheelR1_Audi_A8_1)
  Audi_A8_1/6(SteeringWheel_pivot_Audi_A8_1) -> SteeringWheel_pivot_Audi_A8_1/1(SteeringWheel_pivot_Audi_A8_1)
  Audi_A8_1/7(SteeringColumn_pivot_Audi_A8_1) -> SteeringColumn_pivot_Audi_A8_1/1(SteeringColumn_pivot_Audi_A8_1)
  Audi_A8_1/8(Audi_A8_1_Brake_light_left) -> Audi_A8_1_Brake_light_left/1(Audi_A8_1_Brake_light_left)
  Audi_A8_1/9(Audi_A8_1_Brake_light_right) -> Audi_A8_1_Brake_light_right/1(Audi_A8_1_Brake_light_right)
  Audi_A8_1/10(Audi_A8_1_Indicator_front_left) -> Audi_A8_1_Indicator_front_left/1(Audi_A8_1_Indicator_front_left)
  Audi_A8_1/11(Audi_A8_1_Indicator_rear_left) -> Audi_A8_1_Indicator_rear_left/1(Audi_A8_1_Indicator_rear_left)
  Audi_A8_1/12(Audi_A8_1_Indicator_front_right) -> Audi_A8_1_Indicator_front_right/1(Audi_A8_1_Indicator_front_right)
  Audi_A8_1/13(Audi_A8_1_Indicator_rear_right) -> Audi_A8_1_Indicator_rear_right/1(Audi_A8_1_Indicator_rear_right)
  Sphere_1/1(STATE_Sphere_1_bus) -> STATE_Sphere_1_bus/1(STATE_Sphere_1_bus)
  SELF_Sphere_1/1(SELF_Sphere_1) -> Sphere_1/1(SELF_Sphere_1)
  TrafficLightRoadSideNL_1/1(TrafficLightRoadSideNL_1_Red) -> TrafficLightRoadSideNL_1_Red/1(TrafficLightRoadSideNL_1_Red)
  TrafficLightRoadSideNL_1/2(TrafficLightRoadSideNL_1_Orange) -> TrafficLightRoadSideNL_1_Orange/1(TrafficLightRoadSideNL_1_Orange)
  TrafficLightRoadSideNL_1/3(TrafficLightRoadSideNL_1_Green) -> TrafficLightRoadSideNL_1_Green/1(TrafficLightRoadSideNL_1_Green)
  TrafficLightRoadSideNL_2/1(TrafficLightRoadSideNL_2_Red) -> TrafficLightRoadSideNL_2_Red/1(TrafficLightRoadSideNL_2_Red)
  TrafficLightRoadSideNL_2/2(TrafficLightRoadSideNL_2_Orange) -> TrafficLightRoadSideNL_2_Orange/1(TrafficLightRoadSideNL_2_Orange)
  TrafficLightRoadSideNL_2/3(TrafficLightRoadSideNL_2_Green) -> TrafficLightRoadSideNL_2_Green/1(TrafficLightRoadSideNL_2_Green)
  TrafficLightRoadSideNL_3/1(TrafficLightRoadSideNL_3_Red) -> TrafficLightRoadSideNL_3_Red/1(TrafficLightRoadSideNL_3_Red)
  TrafficLightRoadSideNL_3/2(TrafficLightRoadSideNL_3_Orange) -> TrafficLightRoadSideNL_3_Orange/1(TrafficLightRoadSideNL_3_Orange)
  TrafficLightRoadSideNL_3/3(TrafficLightRoadSideNL_3_Green) -> TrafficLightRoadSideNL_3_Green/1(TrafficLightRoadSideNL_3_Green)
  TrafficLightRoadSideNL_4/1(TrafficLightRoadSideNL_4_Red) -> TrafficLightRoadSideNL_4_Red/1(TrafficLightRoadSideNL_4_Red)
  TrafficLightRoadSideNL_4/2(TrafficLightRoadSideNL_4_Orange) -> TrafficLightRoadSideNL_4_Orange/1(TrafficLightRoadSideNL_4_Orange)
  TrafficLightRoadSideNL_4/3(TrafficLightRoadSideNL_4_Green) -> TrafficLightRoadSideNL_4_Green/1(TrafficLightRoadSideNL_4_Green)
